simulink model "PMSM_Drive_custom_pwm_discrete_HIL_extension"  (R2019b)
settings: Solver=VariableStepAuto  StartTime=0.0  StopTime=1.5  MaxStep=1e-6  RelTol=1e-3
undefined symbols (not defined in the file): Apd, f_sw, In, Tid, U_DC
libraries: coordinate_transformations x4, simulink x2, controllers x1, PE_components x1
settings Model: SimulationMode=accelerator  Creator=kissd  LastModifiedBy=kissd

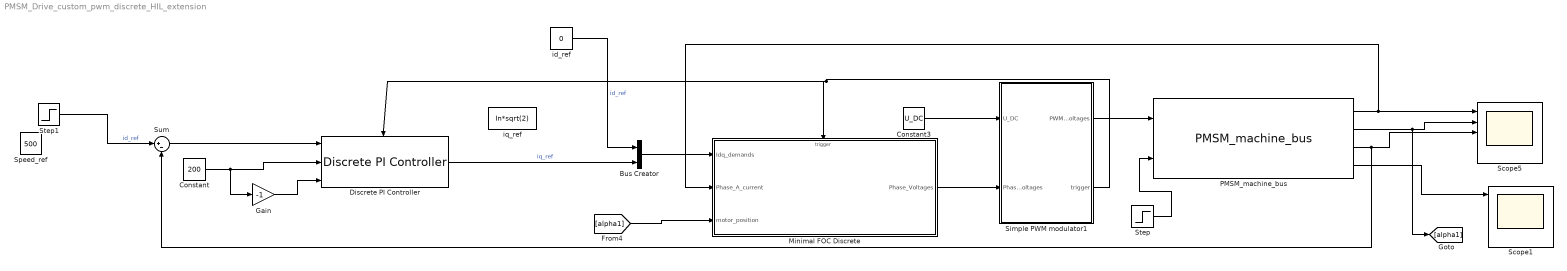
== system PMSM_Drive_custom_pwm_discrete_HIL_extension ==
  Bus Creator : BusCreator  Inputs=2
  Constant : Constant  Value=200
  Constant3 : Constant  Value=U_DC
  Discrete PI Controller : controllers/Discrete PI Controller  Apd=Apd_speed  Tid=Tid_speed  fs=f_sw
  Gain : Gain  Gain=-1
  Minimal FOC Discrete : Subsystem  AncestorBlock=controllers/Minimal FOC Discrete
  PMSM_machine_bus : PE_components/PMSM_machine_bus  SystemSampleTime=-1  Latency=0  AutoFrameSizeCalculation=off
  Scope1 : Scope  NumInputPorts=5
  Scope5 : Scope  NumInputPorts=5
  Simple PWM modulator1 : Subsystem  AncestorBlock=controllers/Simple PWM modulator
  Speed_ref : Constant  Value=500
  Step : Step  Time=0.5  After=60  SampleTime=0
  Step1 : Step  Time=0.75  Before=500  After=1000  SampleTime=0
  Sum : Sum  Inputs=|+-
  id_ref : Constant  Value=0
  iq_ref : Constant  Value=In*sqrt(2)
  wires:
  Constant3/1 -> Simple PWM modulator1/1(U_DC)
  id_ref/1 -> Bus Creator/1  "id_ref"
  Discrete PI Controller/1 -> Bus Creator/2  "iq_ref"
  [alpha1] -> Minimal FOC Discrete/3(motor_position)
  Minimal FOC Discrete/1(Phase_Voltages) -> Simple PWM modulator1/2(Phase_Voltages)
  Simple PWM modulator1/2(trigger) -> Discrete PI Controller/Trigger, Minimal FOC Discrete/Trigger
  Bus Creator/1 -> Minimal FOC Discrete/1(Idq_demands)
  Simple PWM modulator1/1(PWM_Voltages) -> PMSM_machine_bus/1
  PMSM_machine_bus/1 -> Minimal FOC Discrete/2(Phase_A_current), Scope5/1
  PMSM_machine_bus/2 -> Scope5/2, [alpha1]
  PMSM_machine_bus/3 -> Scope5/3, Sum/2
  PMSM_machine_bus/4 -> Scope1/1
  Step1/1 -> Sum/1  "id_ref"
  Sum/1 -> Discrete PI Controller/1
  Constant/1 -> Gain/1, Discrete PI Controller/2
  Gain/1 -> Discrete PI Controller/3
  Step/1 -> PMSM_machine_bus/2

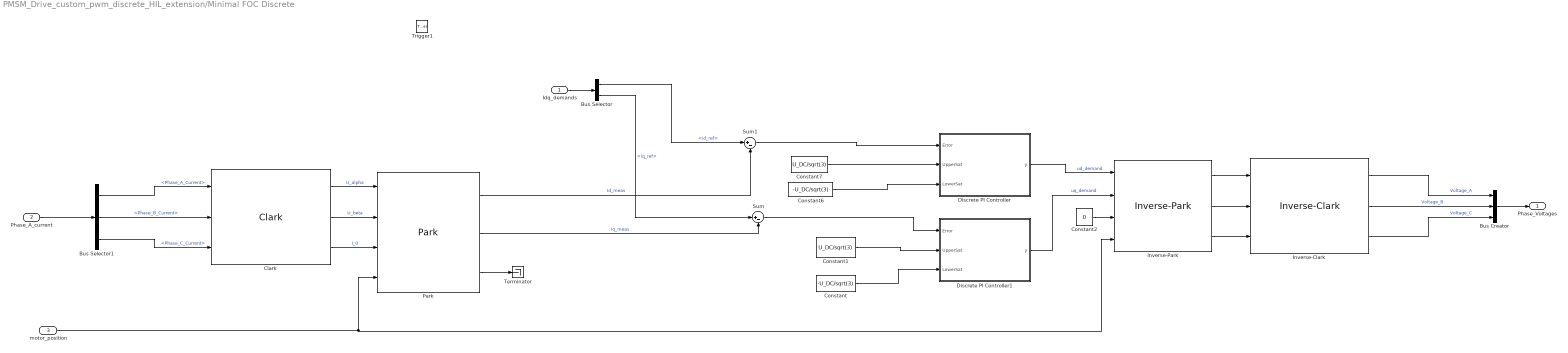
== system PMSM_Drive_custom_pwm_discrete_HIL_extension/Minimal FOC Discrete ==
  Idq_demands : Inport
  Phase_A_current : Inport  Port=2
  motor_position : Inport  Port=3
  Trigger1 : TriggerPort  TriggerType=either  VariantControl=Variant  PortDimensions=1
  Bus Creator : BusCreator  Inputs=3
  Bus Selector : BusSelector  OutputSignals=id_ref,iq_ref
  Bus Selector1 : BusSelector  OutputSignals=Phase_A_Current,Phase_B_Current,Phase_C_Current
  Clark : coordinate_transformations/Clark  SystemSampleTime=-1  Latency=0  AutoFrameSizeCalculation=off
  Constant : Constant  Value=-U_DC/sqrt(3)
  Constant1 : Constant  Value=U_DC/sqrt(3)
  Constant2 : Constant  Value=0
  Constant6 : Constant  Value=-U_DC/sqrt(3)
  Constant7 : Constant  Value=U_DC/sqrt(3)
  Discrete PI Controller : Subsystem  AncestorBlock=controllers/Discrete PI Controller  mask(Continous PI Controller){Apd=Apd, Tid=Tid, fs=f_sw}
      mask prompts: Apd "Proprotional Gain"; Tid "Integration Time"; fs "fsw"
      mask help: Continous PI Controller description.
  Discrete PI Controller1 : Subsystem  AncestorBlock=controllers/Discrete PI Controller  mask(Continous PI Controller){Apd=Apd, Tid=Tid, fs=f_sw}
      mask prompts: Apd "Proprotional Gain"; Tid "Integration Time"; fs "fsw"
      mask help: Continous PI Controller description.
  Inverse-Clark : coordinate_transformations/Inverse-Clark  SystemSampleTime=-1  Latency=0  AutoFrameSizeCalculation=off
  Inverse-Park : coordinate_transformations/Inverse-Park  SystemSampleTime=-1  Latency=0  AutoFrameSizeCalculation=off
  Park : coordinate_transformations/Park  SystemSampleTime=-1  Latency=0  AutoFrameSizeCalculation=off
  Sum : Sum  Inputs=|+-
  Sum1 : Sum  Inputs=|+-
  Terminator : Terminator
  Phase_Voltages : Outport
  wires:
  Discrete PI Controller1/1(y) -> Inverse-Park/2  "uq_demand"
  Inverse-Park/2 -> Inverse-Clark/2
  Inverse-Park/3 -> Inverse-Clark/3
  Park/2 -> Sum/2  "Iq_meas"
  Constant7/1 -> Discrete PI Controller/2(UpperSat)
  Clark/1 -> Park/1  "U_alpha"
  Inverse-Clark/3 -> Bus Creator/3  "Voltage_C"
  Constant1/1 -> Discrete PI Controller1/2(UpperSat)
  Sum/1 -> Discrete PI Controller1/1(Error)
  Inverse-Park/1 -> Inverse-Clark/1
  Constant6/1 -> Discrete PI Controller/3(LowerSat)
  motor_position/1 -> Park/4, Inverse-Park/4
  Park/1 -> Sum1/2  "Id_meas"
  Discrete PI Controller/1(y) -> Inverse-Park/1  "ud_demand"
  Constant/1 -> Discrete PI Controller1/3(LowerSat)
  Sum1/1 -> Discrete PI Controller/1(Error)
  Clark/2 -> Park/2  "U_beta"
  Bus Selector/2 -> Sum/1  "<iq_ref>"
  Clark/3 -> Park/3  "I_0"
  Park/3 -> Terminator/1
  Inverse-Clark/2 -> Bus Creator/2  "Voltage_B"
  Bus Selector/1 -> Sum1/1  "<id_ref>"
  Inverse-Clark/1 -> Bus Creator/1  "Voltage_A"
  Phase_A_current/1 -> Bus Selector1/1
  Constant2/1 -> Inverse-Park/3
  Idq_demands/1 -> Bus Selector/1
  Bus Creator/1 -> Phase_Voltages/1
  Bus Selector1/2 -> Clark/2  "<Phase_B_Current>"
  Bus Selector1/1 -> Clark/1  "<Phase_A_Current>"
  Bus Selector1/3 -> Clark/3  "<Phase_C_Current>"

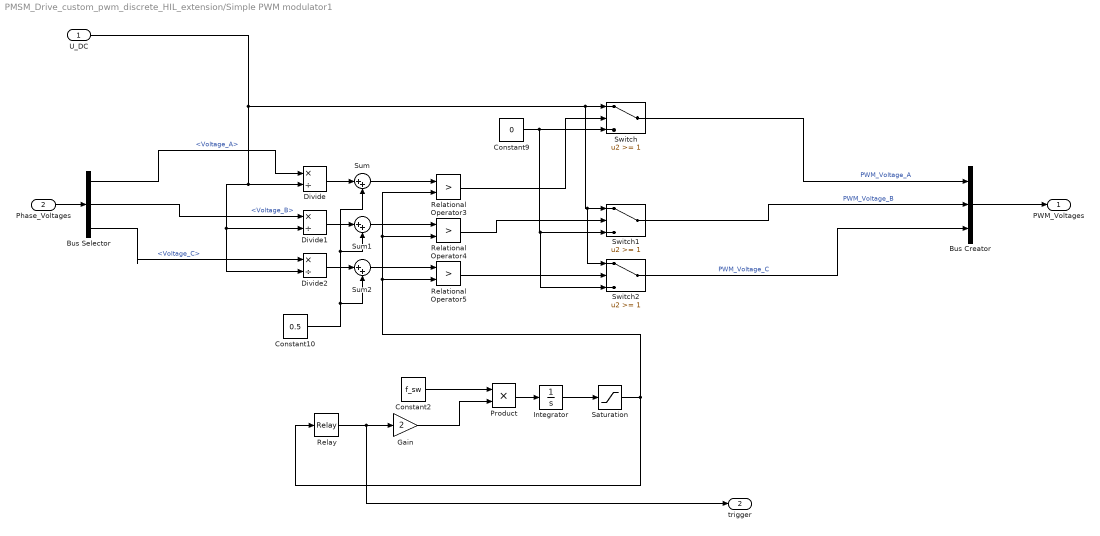
== system PMSM_Drive_custom_pwm_discrete_HIL_extension/Simple PWM modulator1 ==
  U_DC : Inport
  Phase_Voltages : Inport  Port=2
  Bus Creator : BusCreator  Inputs=3
  Bus Selector : BusSelector  OutputSignals=Voltage_A,Voltage_B,Voltage_C
  Constant10 : Constant  Value=0.5
  Constant2 : Constant  Value=f_sw
  Constant9 : Constant  Value=0
  Divide : Product  Inputs=*/
  Divide1 : Product  Inputs=*/
  Divide2 : Product  Inputs=*/
  Gain : Gain  Gain=2
  Integrator : Integrator
  Product : Product
  Relational Operator3 : RelationalOperator  Operator=>  OutDataTypeStr=boolean  RndMeth=Simplest
  Relational Operator4 : RelationalOperator  Operator=>  OutDataTypeStr=boolean  RndMeth=Simplest
  Relational Operator5 : RelationalOperator  Operator=>  OutDataTypeStr=boolean  RndMeth=Simplest
  Relay : Relay  OnSwitchValue=1  OffSwitchValue=0  OnOutputValue=-1  OffOutputValue=1
  Saturation : Saturate  UpperLimit=1  LowerLimit=0
  Sum : Sum  Inputs=|++
  Sum1 : Sum  Inputs=|++
  Sum2 : Sum  Inputs=|++
  Switch : Switch  Threshold=1
  Switch1 : Switch  Threshold=1
  Switch2 : Switch  Threshold=1
  PWM_Voltages : Outport
  trigger : Outport  Port=2
  wires:
  Constant2/1 -> Product/1
  Sum1/1 -> Relational Operator4/1
  Product/1 -> Integrator/1
  Relational Operator5/1 -> Switch2/2
  Integrator/1 -> Saturation/1
  Divide1/1 -> Sum1/1
  Saturation/1 -> Relational Operator3/2, Relational Operator4/2, Relational Operator5/2, Relay/1
  Relay/1 -> trigger/1, Gain/1
  Constant10/1 -> Sum2/2, Sum1/2, Sum/2
  Relational Operator3/1 -> Switch/2
  Switch/1 -> Bus Creator/1  "PWM_Voltage_A"
  Bus Selector/2 -> Divide1/1  "<Voltage_B>"
  Switch2/1 -> Bus Creator/3  "PWM_Voltage_C"
  Constant9/1 -> Switch2/3, Switch1/3, Switch/3
  Relational Operator4/1 -> Switch1/2
  Gain/1 -> Product/2
  Sum/1 -> Relational Operator3/1
  Divide2/1 -> Sum2/1
  Divide/1 -> Sum/1
  Sum2/1 -> Relational Operator5/1
  Bus Selector/3 -> Divide2/1  "<Voltage_C>"
  Bus Selector/1 -> Divide/1  "<Voltage_A>"
  Switch1/1 -> Bus Creator/2  "PWM_Voltage_B"
  U_DC/1 -> Switch2/1, Switch1/1, Switch/1, Divide2/2, Divide1/2, Divide/2
  Phase_Voltages/1 -> Bus Selector/1
  Bus Creator/1 -> PWM_Voltages/1

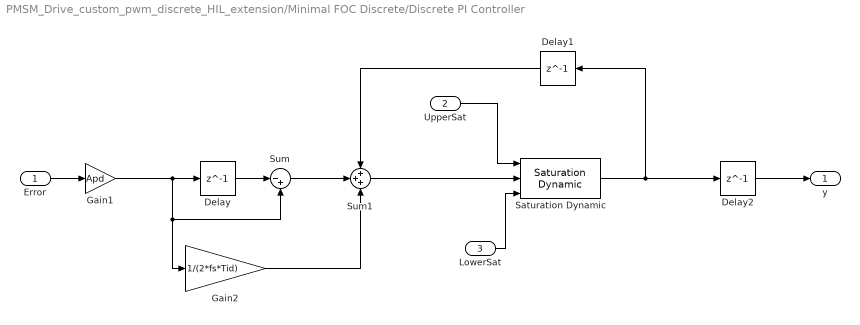
== system PMSM_Drive_custom_pwm_discrete_HIL_extension/Minimal FOC Discrete/Discrete PI Controller ==
  Error : Inport
  UpperSat : Inport  Port=2
  LowerSat : Inport  Port=3
  Delay : Delay  DelayLength=1
  Delay1 : Delay  DelayLength=1
  Delay2 : Delay  DelayLength=1
  Gain1 : Gain  Gain=Apd
  Gain2 : Gain  Gain=1/(2*fs*Tid)
  Saturation Dynamic : simulink/Discontinuities/Saturation Dynamic  OutMin=[]  OutMax=[]  OutDataTypeStr=Inherit: Same as second input  OutDataType=fixdt(1, 16)  OutScaling=2^-10  DoSatur=off
  Sum : Sum  Inputs=|-+
  Sum1 : Sum  Inputs=+++
  y : Outport
  wires:
  Delay2/1 -> y/1
  Delay1/1 -> Sum1/1
  Gain2/1 -> Sum1/3
  Sum/1 -> Sum1/2
  Delay/1 -> Sum/1
  LowerSat/1 -> Saturation Dynamic/3
  UpperSat/1 -> Saturation Dynamic/1
  Saturation Dynamic/1 -> Delay2/1, Delay1/1
  Sum1/1 -> Saturation Dynamic/2
  Gain1/1 -> Delay/1, Sum/2, Gain2/1
  Error/1 -> Gain1/1

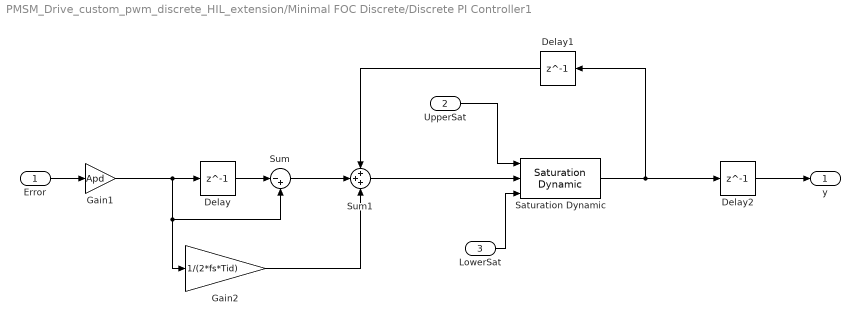
== system PMSM_Drive_custom_pwm_discrete_HIL_extension/Minimal FOC Discrete/Discrete PI Controller1 ==
  Error : Inport
  UpperSat : Inport  Port=2
  LowerSat : Inport  Port=3
  Delay : Delay  DelayLength=1
  Delay1 : Delay  DelayLength=1
  Delay2 : Delay  DelayLength=1
  Gain1 : Gain  Gain=Apd
  Gain2 : Gain  Gain=1/(2*fs*Tid)
  Saturation Dynamic : simulink/Discontinuities/Saturation Dynamic  OutMin=[]  OutMax=[]  OutDataTypeStr=Inherit: Same as second input  OutDataType=fixdt(1, 16)  OutScaling=2^-10  DoSatur=off
  Sum : Sum  Inputs=|-+
  Sum1 : Sum  Inputs=+++
  y : Outport
  wires:
  Delay2/1 -> y/1
  Delay1/1 -> Sum1/1
  Gain2/1 -> Sum1/3
  Sum/1 -> Sum1/2
  Delay/1 -> Sum/1
  LowerSat/1 -> Saturation Dynamic/3
  UpperSat/1 -> Saturation Dynamic/1
  Saturation Dynamic/1 -> Delay2/1, Delay1/1
  Sum1/1 -> Saturation Dynamic/2
  Gain1/1 -> Delay/1, Sum/2, Gain2/1
  Error/1 -> Gain1/1
